simulink model "Evaporator"  (R2016a)
settings: Solver=ode1  StartTime=0.0  StopTime=TimeS  FixedStep=Ts  RelTol=1e-3
values from neighbouring files (symbols this model uses):
  CIf = [Mw0f;Mi0f;Mc0f;Ms0f;T0f]    [SS_Estimator_error_bound.m]
  M_vapor = 1.34    [SS_Estimator_error_bound.m]
  Mc0 = p.cc_o*MTo    [SS_Estimator_error_bound.m]
  Mi0 = double(Sol.Mi0)    [SS_Estimator_error_bound.m]
  Ms0 = double(Sol.Ms0)    [SS_Estimator_error_bound.m]
  Mw0 = double(Sol.Mw0)    [SS_Estimator_error_bound.m]
  T0 = p.T0    [SS_Estimator_error_bound.m]
  ts = 1    [PID_Digital4.m]    (also in SS_Estimator_error_bound.m = 30; UKF_SS.m = 30)
  Ts = 30    [SS_Estimator_error_bound.m]
  ts2 = 30    [SS_Estimator_error_bound.m]    (also in UKF_SS.m)
undefined symbols (not defined in the file or in its folder): arma_Pxe, UKF_SS
libraries: dspsrcs4 x2
settings Model: Creator=Usuario  LastModifiedBy=humbe

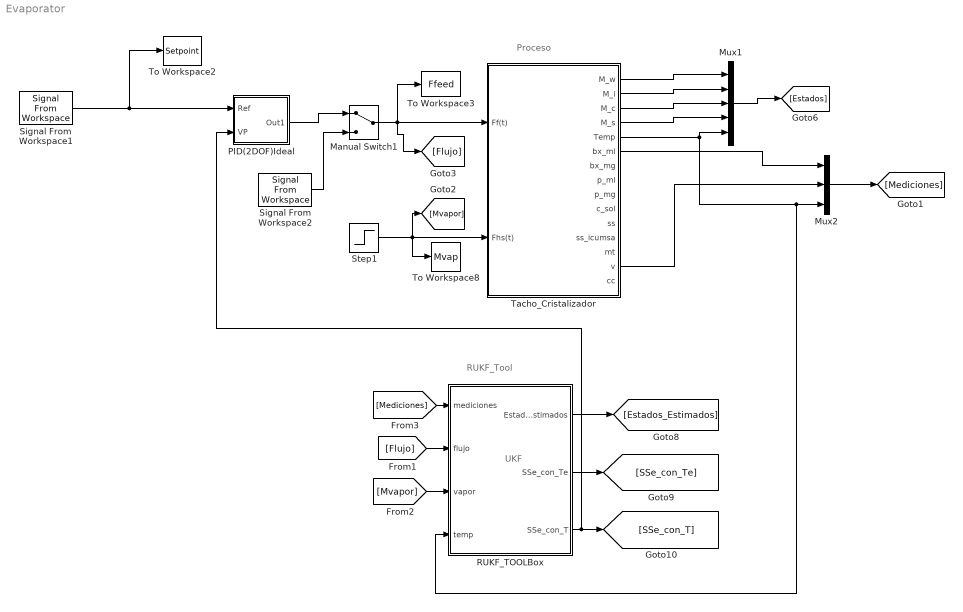
== system Evaporator ==
  note: Proceso
  note: RUKF_Tool
  note: UKF
  Manual Switch1 : ManualSwitch
  Mux1 : Mux  Inputs=5
  Mux2 : Mux  Inputs=3
  PID(2DOF)Ideal : Subsystem
  RUKF_TOOLBox : Subsystem
  Signal From Workspace1 : dspsrcs4/Signal From Workspace  X=Ref_ss  Ts=Ts  nsamps=1  OutputAfterFinalValue=Setting to zero  ignoreOrWarnInputAndFrameLengths=off  OutputFrames=off
  Signal From Workspace2 : dspsrcs4/Signal From Workspace  X=Acc_ctrl  Ts=Ts  nsamps=1  OutputAfterFinalValue=Setting to zero  ignoreOrWarnInputAndFrameLengths=off  OutputFrames=off
  Step1 : Step  Time=0  Before=M_vapor  After=M_vapor  SampleTime=Ts
  Tacho_Cristalizador : Subsystem
  To Workspace2 : ToWorkspace  VariableName=Setpoint  SaveFormat=Timeseries  SampleTime=-1
  To Workspace3 : ToWorkspace  VariableName=Ffeed  SaveFormat=Timeseries  SampleTime=-1
  To Workspace8 : ToWorkspace  VariableName=Mvap  SaveFormat=Timeseries  SampleTime=Ts
  wires:
  Step1/1 -> [Mvapor], Tacho_Cristalizador/2(Fhs(t)), To Workspace8/1
  Tacho_Cristalizador/5(Temp) -> Mux1/5, RUKF_TOOLBox/4(temp), Mux2/3
  Tacho_Cristalizador/4(M_s) -> Mux1/4
  Tacho_Cristalizador/3(M_c) -> Mux1/3
  Tacho_Cristalizador/2(M_i) -> Mux1/2
  Tacho_Cristalizador/1(M_w) -> Mux1/1
  Mux1/1 -> [Estados]
  Mux2/1 -> [Mediciones]
  Tacho_Cristalizador/6(bx_ml) -> Mux2/1
  Tacho_Cristalizador/14(v) -> Mux2/2
  Signal From Workspace2/1 -> Manual Switch1/2
  Signal From Workspace1/1 -> PID(2DOF)Ideal/1(Ref), To Workspace2/1
  [Mediciones] -> RUKF_TOOLBox/1(mediciones)
  [Flujo] -> RUKF_TOOLBox/2(flujo)
  [Mvapor] -> RUKF_TOOLBox/3(vapor)
  RUKF_TOOLBox/1(Estados_estimados) -> [Estados_Estimados]
  RUKF_TOOLBox/2(SSe_con_Te) -> [SSe_con_Te]
  RUKF_TOOLBox/3(SSe_con_T) -> PID(2DOF)Ideal/2(VP), [SSe_con_T]
  PID(2DOF)Ideal/1(Out1) -> Manual Switch1/1
  Manual Switch1/1 -> [Flujo], To Workspace3/1, Tacho_Cristalizador/1(Ff(t))

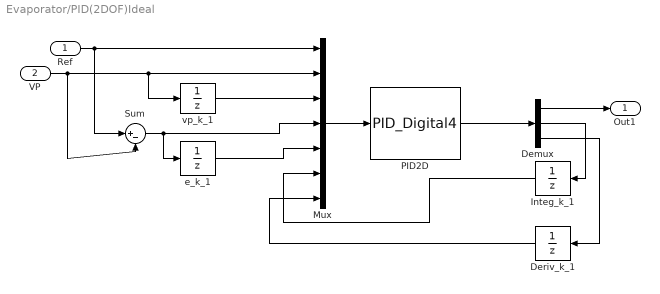
== system Evaporator/PID(2DOF)Ideal ==
  Ref : Inport
  VP : Inport  Port=2
  Demux : Demux  Outputs=3
  Deriv_k_1 : UnitDelay  SampleTime=ts2
  Integ_k_1 : UnitDelay  SampleTime=ts2
  Mux : Mux  Inputs=7
  PID2D : MATLABFcn  MATLABFcn=PID_Digital4  OutputDimensions=3  Output1D=off  SampleTime=ts2
  Sum : Sum  Inputs=|+-
  e_k_1 : UnitDelay  SampleTime=ts2
  "vp_k_1 " : UnitDelay  SampleTime=ts2
  Out1 : Outport
  wires:
  Mux/1 -> PID2D/1
  Ref/1 -> Mux/1, Sum/1
  VP/1 -> Sum/2, "vp_k_1 "/1, Mux/2
  "vp_k_1 "/1 -> Mux/3
  Sum/1 -> e_k_1/1, Mux/4
  e_k_1/1 -> Mux/5
  PID2D/1 -> Demux/1
  Demux/1 -> Out1/1
  Demux/2 -> Integ_k_1/1
  Demux/3 -> Deriv_k_1/1
  Integ_k_1/1 -> Mux/6
  Deriv_k_1/1 -> Mux/7

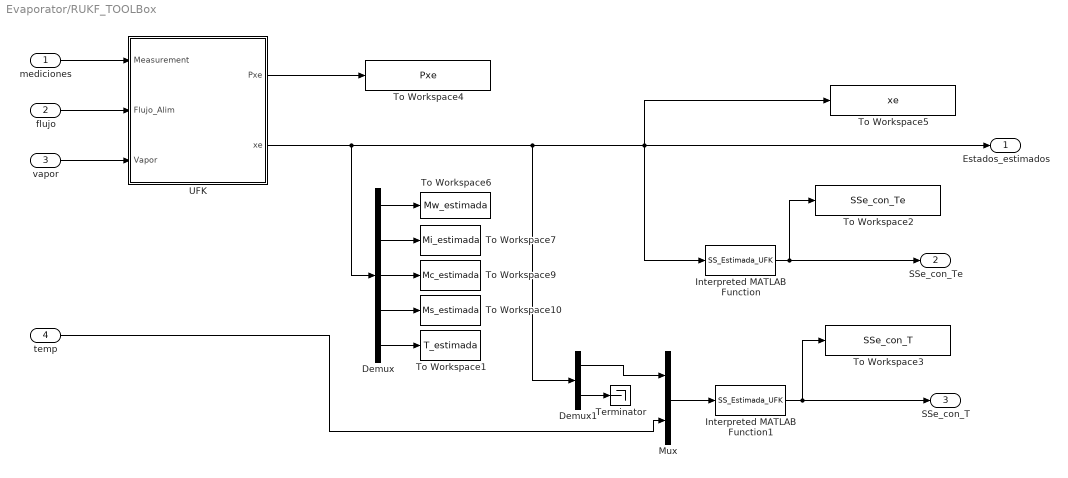
== system Evaporator/RUKF_TOOLBox ==
  mediciones : Inport
  flujo : Inport  Port=2
  vapor : Inport  Port=3
  temp : Inport  Port=4
  Demux : Demux  Outputs=5
  Demux1 : Demux  Outputs=[4,1]
  Interpreted MATLAB Function : MATLABFcn  MATLABFcn=SS_Estimada_UFK  OutputDimensions=1
  Interpreted MATLAB Function1 : MATLABFcn  MATLABFcn=SS_Estimada_UFK  OutputDimensions=1
  Mux : Mux  Inputs=2
  Terminator : Terminator
  To Workspace1 : ToWorkspace  VariableName=T_estimada  SaveFormat=Timeseries  SampleTime=ts
  To Workspace10 : ToWorkspace  VariableName=Ms_estimada  SaveFormat=Timeseries  SampleTime=Ts
  To Workspace2 : ToWorkspace  VariableName=SSe_con_Te  SaveFormat=Timeseries  SampleTime=-1
  To Workspace3 : ToWorkspace  VariableName=SSe_con_T  SaveFormat=Timeseries  SampleTime=-1
  To Workspace4 : ToWorkspace  VariableName=Pxe  SaveFormat=Timeseries  SampleTime=-1
  To Workspace5 : ToWorkspace  VariableName=xe  SaveFormat=Timeseries  SampleTime=-1
  To Workspace6 : ToWorkspace  VariableName=Mw_estimada  SaveFormat=Timeseries  SampleTime=Ts
  To Workspace7 : ToWorkspace  VariableName=Mi_estimada  SaveFormat=Timeseries  SampleTime=Ts
  To Workspace9 : ToWorkspace  VariableName=Mc_estimada  SaveFormat=Timeseries  SampleTime=Ts
  UFK : Subsystem
  Estados_estimados : Outport
  SSe_con_Te : Outport  Port=2
  SSe_con_T : Outport  Port=3
  wires:
  Mux/1 -> Interpreted MATLAB Function1/1
  Interpreted MATLAB Function1/1 -> SSe_con_T/1, To Workspace3/1
  Demux1/1 -> Mux/1
  Demux1/2 -> Terminator/1
  Demux/5 -> To Workspace1/1
  Demux/4 -> To Workspace10/1
  Demux/3 -> To Workspace9/1
  Demux/2 -> To Workspace7/1
  Demux/1 -> To Workspace6/1
  temp/1 -> Mux/2
  flujo/1 -> UFK/2(Flujo_Alim)
  Interpreted MATLAB Function/1 -> To Workspace2/1, SSe_con_Te/1
  mediciones/1 -> UFK/1(Measurement)
  vapor/1 -> UFK/3(Vapor)
  UFK/2(xe) -> Demux1/1, To Workspace5/1, Interpreted MATLAB Function/1, Estados_estimados/1, Demux/1
  UFK/1(Pxe) -> To Workspace4/1

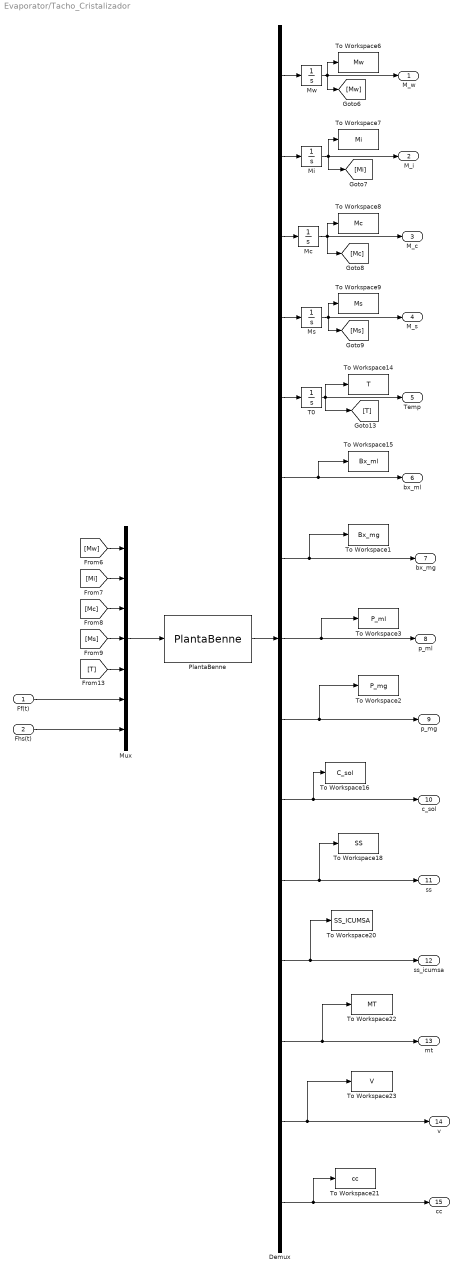
== system Evaporator/Tacho_Cristalizador ==
  Ff(t) : Inport
  Fhs(t) : Inport  Port=2
  Demux : Demux  Outputs=15
  Mc : Integrator  InitialCondition=Mc0
  Mi : Integrator  InitialCondition=Mi0
  Ms : Integrator  InitialCondition=Ms0
  Mux : Mux  Inputs=7
  Mw : Integrator  InitialCondition=Mw0
  PlantaBenne : MATLABFcn  MATLABFcn=PlantaBenne  OutputDimensions=15
  T0 : Integrator  InitialCondition=T0
  To Workspace1 : ToWorkspace  VariableName=Bx_mg  SaveFormat=Timeseries  SampleTime=Ts
  To Workspace14 : ToWorkspace  VariableName=T  SaveFormat=Timeseries  SampleTime=Ts
  To Workspace15 : ToWorkspace  VariableName=Bx_ml  SaveFormat=Timeseries  SampleTime=Ts
  To Workspace16 : ToWorkspace  VariableName=C_sol  SaveFormat=Timeseries  SampleTime=Ts
  To Workspace18 : ToWorkspace  VariableName=SS  SaveFormat=Timeseries  SampleTime=Ts
  To Workspace2 : ToWorkspace  VariableName=P_mg  SaveFormat=Timeseries  SampleTime=Ts
  To Workspace20 : ToWorkspace  VariableName=SS_ICUMSA  SaveFormat=Timeseries  SampleTime=Ts
  To Workspace21 : ToWorkspace  VariableName=cc  SaveFormat=Timeseries  SampleTime=Ts
  To Workspace22 : ToWorkspace  VariableName=MT  SaveFormat=Timeseries  SampleTime=Ts
  To Workspace23 : ToWorkspace  VariableName=V  SaveFormat=Timeseries  SampleTime=Ts
  To Workspace3 : ToWorkspace  VariableName=P_ml  SaveFormat=Timeseries  SampleTime=Ts
  To Workspace6 : ToWorkspace  VariableName=Mw  SaveFormat=Timeseries  SampleTime=Ts
  To Workspace7 : ToWorkspace  VariableName=Mi  SaveFormat=Timeseries  SampleTime=Ts
  To Workspace8 : ToWorkspace  VariableName=Mc  SaveFormat=Timeseries  SampleTime=Ts
  To Workspace9 : ToWorkspace  VariableName=Ms  SaveFormat=Timeseries  SampleTime=Ts
  M_w : Outport
  M_i : Outport  Port=2
  M_c : Outport  Port=3
  M_s : Outport  Port=4
  Temp : Outport  Port=5
  bx_ml : Outport  Port=6
  bx_mg : Outport  Port=7
  p_ml : Outport  Port=8
  p_mg : Outport  Port=9
  c_sol : Outport  Port=10
  ss : Outport  Port=11
  ss_icumsa : Outport  Port=12
  mt : Outport  Port=13
  v : Outport  Port=14
  cc : Outport  Port=15
  wires:
  Mux/1 -> PlantaBenne/1
  Mi/1 -> M_i/1, To Workspace7/1, [Mi]
  Ms/1 -> To Workspace9/1, M_s/1, [Ms]
  Mw/1 -> [Mw], M_w/1, To Workspace6/1
  Mc/1 -> M_c/1, [Mc], To Workspace8/1
  PlantaBenne/1 -> Demux/1
  T0/1 -> [T], Temp/1, To Workspace14/1
  [Mw] -> Mux/1
  [Mi] -> Mux/2
  [Mc] -> Mux/3
  [Ms] -> Mux/4
  [T] -> Mux/5
  Ff(t)/1 -> Mux/6
  Fhs(t)/1 -> Mux/7
  Demux/1 -> Mw/1
  Demux/4 -> Ms/1
  Demux/3 -> Mc/1
  Demux/2 -> Mi/1
  Demux/5 -> T0/1
  Demux/6 -> bx_ml/1, To Workspace15/1
  Demux/7 -> bx_mg/1, To Workspace1/1
  Demux/8 -> p_ml/1, To Workspace3/1
  Demux/9 -> To Workspace2/1, p_mg/1
  Demux/10 -> To Workspace16/1, c_sol/1
  Demux/11 -> To Workspace18/1, ss/1
  Demux/12 -> To Workspace20/1, ss_icumsa/1
  Demux/14 -> v/1, To Workspace23/1
  Demux/15 -> To Workspace21/1, cc/1
  Demux/13 -> To Workspace22/1, mt/1

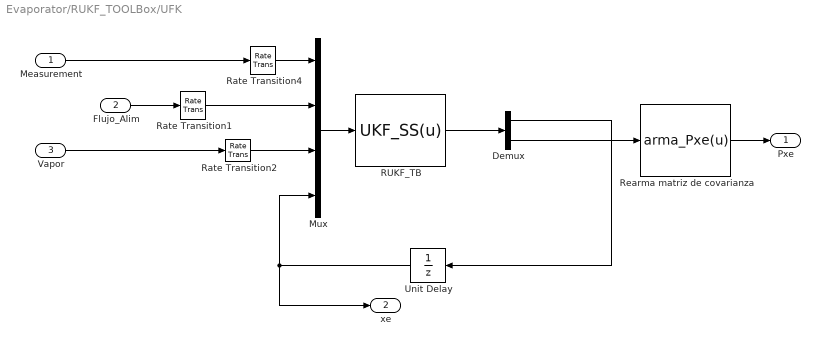
== system Evaporator/RUKF_TOOLBox/UFK ==
  Measurement : Inport
  Flujo_Alim : Inport  Port=2
  Vapor : Inport  Port=3
  Demux : Demux  Outputs=[5,25]
  Mux : Mux
  RUKF_TB : MATLABFcn  MATLABFcn=UKF_SS(u)  OutputDimensions=30  Output1D=off  SampleTime=ts2
  Rate Transition1 : RateTransition  X0=7.7  OutPortSampleTime=ts2
  Rate Transition2 : RateTransition  X0=7.7  OutPortSampleTime=ts2
  Rate Transition4 : RateTransition  X0=7.7  OutPortSampleTime=ts2
  Rearma matriz de covarianza : MATLABFcn  MATLABFcn=arma_Pxe(u)  Output1D=off  SampleTime=ts2
  Unit Delay : UnitDelay  InitialCondition=CIf  SampleTime=ts2
  Pxe : Outport
  xe : Outport  Port=2
  wires:
  Rearma matriz de covarianza/1 -> Pxe/1
  Demux/2 -> Rearma matriz de covarianza/1
  Demux/1 -> Unit Delay/1
  RUKF_TB/1 -> Demux/1
  Vapor/1 -> Rate Transition2/1
  Mux/1 -> RUKF_TB/1
  Rate Transition1/1 -> Mux/2
  Unit Delay/1 -> Mux/4, xe/1
  Flujo_Alim/1 -> Rate Transition1/1
  Rate Transition2/1 -> Mux/3
  Rate Transition4/1 -> Mux/1
  Measurement/1 -> Rate Transition4/1
